simulink model "closed_loop_simulation"  (Simulink 8.1)
settings: Solver=FixedStepDiscrete  StartTime=0.0  StopTime=21.0  FixedStep=0.3  RelTol=1e-3
settings Model: Creator=madwolf  LastModifiedBy=madwolf
settings DataIOCC: SignalLoggingSaveFormat=Dataset
settings OptimizationCC: ExpressionDepthLimit=128
settings DebuggingCC: FcnCallInpInsideContextMsg=EnableAllAsError
settings RTWCC: GenerateReport=on  RTWUseSimCustomCode=on  LaunchReport=on  TargetLang=C++
settings GRTTargetCC: CombineOutputUpdateFcns=on  GRTInterface=off

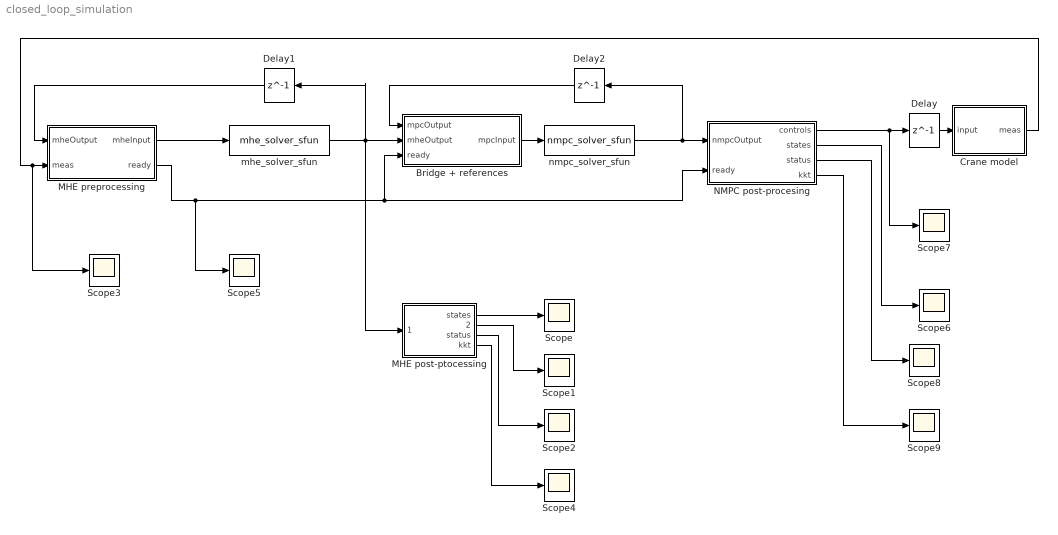
== system closed_loop_simulation ==
  Bridge + references : MATLAB Function  TreatAsAtomicUnit=on
  Crane model : MATLAB Function  TreatAsAtomicUnit=on
  Delay : Delay  DelayLength=1  InitialCondition=0
  Delay1 : Delay  DelayLength=1  InitialCondition=0
  Delay2 : Delay  DelayLength=1  InitialCondition=0
  MHE post-ptocessing : MATLAB Function  TreatAsAtomicUnit=on
  MHE preprocessing : MATLAB Function  TreatAsAtomicUnit=on
  NMPC post-procesing : MATLAB Function  TreatAsAtomicUnit=on
  Scope{,1..9} (10 alike) : Scope
      Scope2 settings: SaveName=ScopeData2
      Scope3 settings: SaveName=ScopeData3
      Scope4 settings: SaveName=mheKktValue
      Scope5 settings: SaveName=ScopeData4
      Scope6 settings: SaveName=ScopeData5
      Scope7 settings: SaveName=ScopeData6
      Scope8 settings: SaveName=ScopeData7
      Scope9 settings: SaveName=ScopeData8
  mhe_solver_sfun : S-Function  FunctionName=mhe_solver_sfun  EnableBusSupport=off  mask(Legacy Function){SFunctionSpec=mhe_solver_wrapper(mheinput u1[1], mheoutput y1[1]), ShowSpec=on}
      mask prompts: ShowSpec "Display function specification"
      mask help:
      | This block allows you to call the legacy functions specified by the following Legacy Code Tool definition:
      | def.SFunctionName = 'mhe_solver_sfun';
      | def.OutputFcnSpec = 'mhe_solver_wrapper(mheinput u1[1], mheoutput y1[1])';
      | def.HeaderFiles = {'mhe_common.h', 'mhe_solver_sfunction.h'};
      | def.SourceFiles = {'qpoases/SRC/QProblem.cpp', 'qpoases/SRC/QProblemB.cpp', 'qpoases/SRC/Bounds.cpp', 'qpoases/SRC/Constraints.cpp', 'qpoases/SRC/SubjectTo.cpp', 'qpoases/SRC/Indexlist.cpp', 'qpoases/SRC/CyclingManager.cpp', 'qpoases/SRC/Utils.cpp', 'qpoases/SRC/MessageHandling.cpp', 'qpoases/SRC/EXTRAS/SolutionAnalysis.cpp', 'mhe_solver.c', 'mhe_integrator.c', 'mhe_auxiliary_functions.c', 'mhe_qpoases_interface.cpp', 'mhe_solver_sfunction.c'};
      | def.IncPaths = {'qpoases', 'qpoases/INCLUDE', 'qpoases/SRC'};
      | def.Options.language = 'C++';
      mask Help: <p>This block was generated automatically by the Legacy Code Tool. For detailed help on this tool, call<a href="matlab:legacy_code('help')"> legacy_code('help')</a>.</p>
      mask Callback ShowSpec:
      | if strcmp(get_param(gcbh, 'ShowSpec'), 'on')
      |   set_param(gcbh, 'MaskDisplay', sprintf('fprintf(''%s'');', get_param(gcbh, 'SFunctionSpec')));
      | else
      |   set_param(gcbh, 'MaskDisplay', sprintf('fprintf(''%s'');', get_param(gcbh, 'FunctionName')));
      | end
      mask Display: fprintf('mhe_solver_wrapper(mheinput u1[1], mheoutput y1[1])');
  nmpc_solver_sfun : S-Function  FunctionName=nmpc_solver_sfun  EnableBusSupport=off  mask(Legacy Function){SFunctionSpec=nmpc_solver_wrapper(nmpcinput u1[1], nmpcoutput y1[1]), ShowSpec=on}
      mask prompts: ShowSpec "Display function specification"
      mask help:
      | This block allows you to call the legacy functions specified by the following Legacy Code Tool definition:
      | def.SFunctionName = 'nmpc_solver_sfun';
      | def.OutputFcnSpec = 'nmpc_solver_wrapper(nmpcinput u1[1], nmpcoutput y1[1])';
      | def.HeaderFiles = {'nmpc_common.h', 'nmpc_solver_sfunction.h'};
      | def.SourceFiles = {'qpoases/SRC/QProblem.cpp', 'qpoases/SRC/QProblemB.cpp', 'qpoases/SRC/Bounds.cpp', 'qpoases/SRC/Constraints.cpp', 'qpoases/SRC/SubjectTo.cpp', 'qpoases/SRC/Indexlist.cpp', 'qpoases/SRC/CyclingManager.cpp', 'qpoases/SRC/Utils.cpp', 'qpoases/SRC/MessageHandling.cpp', 'qpoases/SRC/EXTRAS/SolutionAnalysis.cpp', 'nmpc_solver.c', 'nmpc_integrator.c', 'nmpc_auxiliary_functions.c', 'nmpc_qpoases_interface.cpp', 'nmpc_solver_sfunction.c'};
      | def.IncPaths = {'qpoases', 'qpoases/INCLUDE', 'qpoases/SRC'};
      | def.Options.language = 'C++';
      mask Help: <p>This block was generated automatically by the Legacy Code Tool. For detailed help on this tool, call<a href="matlab:legacy_code('help')"> legacy_code('help')</a>.</p>
      mask Callback ShowSpec:
      | if strcmp(get_param(gcbh, 'ShowSpec'), 'on')
      |   set_param(gcbh, 'MaskDisplay', sprintf('fprintf(''%s'');', get_param(gcbh, 'SFunctionSpec')));
      | else
      |   set_param(gcbh, 'MaskDisplay', sprintf('fprintf(''%s'');', get_param(gcbh, 'FunctionName')));
      | end
      mask Display: fprintf('nmpc_solver_wrapper(nmpcinput u1[1], nmpcoutput y1[1])');
  wires:
  nmpc_solver_sfun/1 -> Delay2/1, NMPC post-procesing/1(nmpcOutput)
  Bridge + references/1(mpcInput) -> nmpc_solver_sfun/1
  mhe_solver_sfun/1 -> MHE post-ptocessing/1(mheOutput), Delay1/1, Bridge + references/2(mheOutput)
  MHE preprocessing/1(mheInput) -> mhe_solver_sfun/1
  MHE preprocessing/2(ready) -> Scope5/1, Bridge + references/3(ready), NMPC post-procesing/2(ready)
  Delay1/1 -> MHE preprocessing/1(mheOutput)
  Delay2/1 -> Bridge + references/1(mpcOutput)
  MHE post-ptocessing/2(control) -> Scope1/1
  MHE post-ptocessing/1(states) -> Scope/1
  MHE post-ptocessing/3(status) -> Scope2/1
  MHE post-ptocessing/4(kkt) -> Scope4/1
  NMPC post-procesing/1(controls) -> Scope7/1, Delay/1
  Crane model/1(meas) -> Scope3/1, MHE preprocessing/2(meas)
  Delay/1 -> Crane model/1(input)
  NMPC post-procesing/2(states) -> Scope6/1
  NMPC post-procesing/3(status) -> Scope8/1
  NMPC post-procesing/4(kkt) -> Scope9/1

== matlab function Bridge + references ==
  data: mpcOutput input Bus: nmpcoutput; mheOutput input Bus: mheoutput; mpcInput output Bus: nmpcinput; ready input double
function mpcInput = fcn(mpcOutput, mheOutput, ready)
%#codegen

%% Dimenions
NX = 4;
NU = 1;
% MHE_NY = 3;
% MHE_NYN = 2;

MPC_NY = 5;
MPC_NYN = 4;

% In this case, it is equal for MHE and NMPC.
N = 10;

%% Setup data structures

persistent input
if isempty ( input )
    % Do nothing
    input.control = int32( 10 );
    % Always use integration from the last node for shifting
    input.shifting = int32( 2 );
    % Initialization by a forward simulation.
    input.initialization = int32( 1 );
    
    %%% NOTE: All arrays are 1-D.
    input.data.x = zeros(1, (N + 1) * NX);
    input.data.u = zeros(1, N * NU);
    input.data.y = zeros(1, N * MPC_NY);
    input.data.yN = zeros(1, MPC_NYN);
    
    % Set up the weighting matrices
    eye1 = eye( MPC_NY ) * 1;
    eye5 = eye( MPC_NYN ) * 5;
    
    input.data.W = eye1(:)';
    input.data.WN = eye5(:)';
    
    input.data.x0 = zeros(1, NX);
end;

persistent nmpcStarted
if isempty( nmpcStarted )
    nmpcStarted = 0;
end;

if ready
    % The estimator started spitting some estimates
    
    % Here we read the current state estimate
    input.data.x0 = mheOutput.data.x(N * NX + 1: (N + 1) * NX);
    
    % However, we would like to wait a bit until the estimator converges
    if (nmpcStarted == 0) && (mheOutput.kktValue < 1e-6)
        mheOutput.kktValue
        nmpcStarted = 1;
    end;
    
    % If it converged, enable controller execution
    if nmpcStarted == 1
        % Simple running more
        input.control = int32( 0 );
    end;
else
    % Do nothing
    input.control = int32( 10 );
end;

persistent firstRun
if isempty( firstRun )
    firstRun = 1;
end;

if firstRun == 1
    % Reset the flag. 
    firstRun = 0;
else
    % NOTE: Those guys are first gonna be shifted because of the option
    %       at line 23.
    input.data.x = mpcOutput.data.x;
    input.data.u = mpcOutput.data.u;
end;

%% Output the data structures
mpcInput = input;

== matlab function MHE preprocessing ==
  data: mheOutput input Bus: mheoutput; meas input double; mheInput output Bus: mheinput; ready output boolean
function [mheInput, ready] = fcn(mheOutput, meas)
%#codegen

%% Dimensions, MHE
NX = 4;
NU = 1;
NY = 3;
NYN = 2;
N = 10;

persistent output
if isempty( output )
    % Initially, do not do anything, untill we fill in the measurements
    % buffer
    output.control = int32( 10 );
    % Always use integration from the last node for shifting
    output.shifting = int32( 2 );
    % Initialization by a forward simulation.
    output.initialization = int32( 1 );
    
    %%% NOTE: All arrays are 1-D.
    output.data.x = zeros(1, (N + 1) * NX);
    output.data.u = zeros(1, N * NU);
    output.data.y = zeros(1, N * NY);
    output.data.yN = zeros(1, NYN);
    
    eyeNY = diag(1e-4 ./ [0.01, 0.01, 0.1].^2);
    eyeNYN = diag(1e-4 ./ [0.01, 0.01].^2);
    
    output.data.W = eyeNY(:)';
    output.data.WN = eyeNYN(:)';
end;

persistent runCnt
if isempty( runCnt )
    runCnt = 1;
end;

persistent execReady
if isempty( execReady )
    execReady = 0;
end;

if runCnt < (N + 1)
    % Fill in the measurement buffer, entries 1: N

    output.data.y((runCnt - 1) * NY + 1: runCnt * NY) = meas;
    
    % Initialize solver, measured states, shooting nodes 1: N
    output.data.x((runCnt - 1) * NX + 1) = meas( 1 );
    output.data.x((runCnt - 1) * NX + 3) = meas( 2 );
    
    % MHE is not ready, of course.
    execReady = 0;
    
    % Increment counter
    runCnt = runCnt + 1;
    
elseif runCnt == (N + 1)
    % Initialize measurements on node N + 1,
    output.data.yN = meas(1: 2, 1)';
    % Initialize measured controls on previous node, node N
    output.data.y((N - 1) * NY + 3) = meas(3, 1);
    
    % Initialize measured states on node N _ 1
    output.data.x((runCnt - 1) * NX + 1) = meas( 1 );
    output.data.x((runCnt - 1) * NX + 3) = meas( 2 );
    
    % Simple running more
    output.control = int32( 0 );
    
    % MHE is still not ready, we want to run it once before we use the
    % state estimate.
    execReady = 0;
    
    % Increment the counter.
    runCnt = runCnt + 1;
    
else
    % Shift measurements
    for i = 1: N - 1
        output.data.y((i - 1) * NY + 1: i * NY) = output.data.y(i * NY + 1: (i + 1) * NY);
    end;
    output.data.y((N - 1) * NY + 1: (N - 1) * NY + 2) = output.data.yN;
    
    output.data.yN = meas(1: 2, 1)';
    output.data.y((N - 1) * NY + 3) = meas(3, 1);
    
    % Use previous states and controls (solutions!) for initialization.
    % NOTE: Those guys are first gonna be shifted because of the option
    %       at line 17.
    
    output.data.x = mheOutput.data.x;
    output.data.u = mheOutput.data.u;
    
    output.control = int32( 0 );
    
    % Yeah, we are ready now.
    execReady = 1;
end;

%% Output data
mheInput = output;
ready = execReady;

== matlab function Crane model ==
  data: input input double size=1; meas output double size=3
function meas = fcn(input)
%#codegen

%% Dimensions, model and MHE
NX = 4;
NU = 1;
NY = 3;
NYN = 2;

Ts = 0.3;
Ni = 3;

persistent x0
if isempty( x0 )
    x0 = [2.0, 0, 0, 0]';
end;

persistent state
if isempty( state )
    state = x0;
end;

persistent execMeas
if isempty( execMeas )
    execMeas = zeros(NY, 1);
end;

%% Model integration. Here we use a simple RK4 integrator

h = Ts / Ni;

for i = 1: Ni
    k1 = rhs(input, state           );
    k2 = rhs(input, state + 0.5 * k1);
    k3 = rhs(input, state + 0.5 * k2);
    k4 = rhs(input, state + k3      );
    
    state = state + 1/6 * h * (k1 + 2 * k2 + 2 * k3 + k4);
end;

%% Set measurements

execMeas( 1 ) = state( 1 );
execMeas( 2 ) = state( 3 );
execMeas( 3 ) = input( 1 );

meas = execMeas;

function [xdot] = rhs(u, x)
%#codegen

g = 9.81;
b = 0.2;

xdot = zeros(4, 1);

xdot( 1 ) = x( 2 );
xdot( 2 ) = u;
xdot( 3 ) = x( 4 );
xdot( 4 ) = -g * sin(x( 3 )) - u * cos(x( 3 )) - b * x( 4 );

== matlab function MHE post-ptocessing ==
  data: mheOutput input Bus: mheoutput; states output double; control output double; status output double; kkt output double
function [states,control, status, kkt] = fcn(mheOutput)
%#codegen

%% Dimensions, MHE
NX = 4;
NU = 1;
N = 10;

% The current state estimate.
states = mheOutput.data.x(N * NX + 1: (N + 1) * NX);
% Last estimated controls.
control = mheOutput.data.u(N * NU);
% Status of the QP solver.
status =  mheOutput.status;

if status >= 0
    % Output KKT only is QP solver status is OK.
    kkt = mheOutput.kktValue;
else
    % This can be used for debugging purposes.
    kkt = -1;
end;

== matlab function NMPC post-procesing ==
  data: nmpcOutput input Bus: nmpcoutput; controls output double; states output double; ready input double; status output double; kkt output double
function [controls, states,status, kkt] = fcn(nmpcOutput, ready)
%#codegen

%% Dimensions, NMPC
NX = 4;
NU = 1;

states = nmpcOutput.data.x0;

if ready == 1
    controls = nmpcOutput.data.u( 1 );
else
    controls = 0;
end;

kkt = nmpcOutput.kktValue;
status = nmpcOutput.status;
